simulink model "example"  (R2021b)
settings: Solver=VariableStepAuto  StartTime=0.0  StopTime=10.0  RelTol=1e-3
settings Model: Creator=Studenci  LastModifiedBy=Studenci

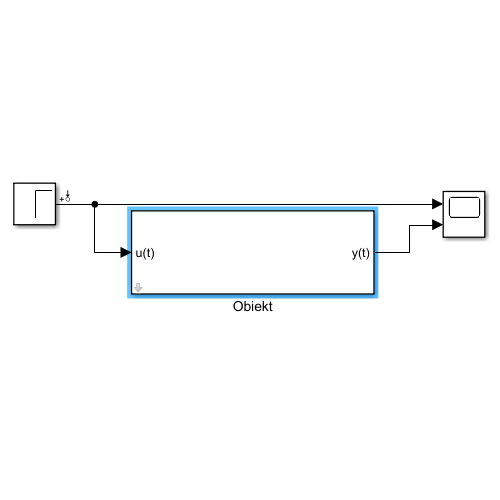
[thumbnail: Simulink's stored preview of the top-level diagram]
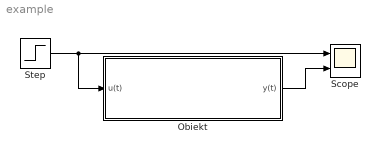
== system example ==
  Obiekt : Subsystem  mask{wn=1, zeta=0.5}
      mask prompts: wn "wn - częstotliwość drgań własnych"; zeta "zeta - współczynnik tłumienia"
  Scope : Scope  NumInputPorts=2
  Step : Step  Time=0  SampleTime=0
  wires:
  Step/1 -> Obiekt/1(u(t)), Scope/1
  Obiekt/1(y(t)) -> Scope/2

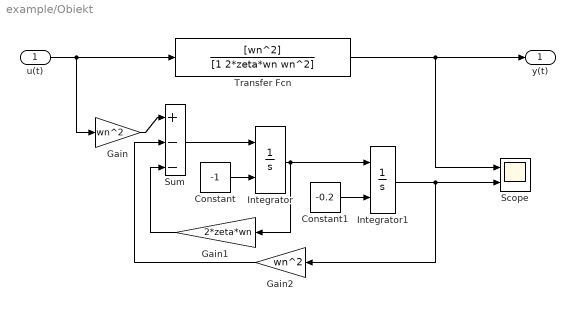
== system example/Obiekt ==
  u(t) : Inport
  Constant : Constant  Value=-1
  Constant1 : Constant  Value=-0.2
  Gain : Gain  Gain=wn^2
  Gain1 : Gain  Gain=2*zeta*wn
  Gain2 : Gain  Gain=wn^2
  Integrator : Integrator  InitialConditionSource=external
  Integrator1 : Integrator  InitialConditionSource=external
  Scope : Scope  NumInputPorts=2
  Sum : Sum  Inputs=|+--
  Transfer Fcn : TransferFcn  Numerator=[wn^2]  Denominator=[1 2*zeta*wn wn^2]
  y(t) : Outport
  wires:
  Transfer Fcn/1 -> Scope/1, y(t)/1
  u(t)/1 -> Transfer Fcn/1, Gain/1
  Gain/1 -> Sum/1
  Constant/1 -> Integrator/2
  Sum/1 -> Integrator/1
  Integrator/1 -> Gain1/1, Integrator1/1
  Constant1/1 -> Integrator1/2
  Integrator1/1 -> Gain2/1, Scope/2
  Gain1/1 -> Sum/3
  Gain2/1 -> Sum/2
